simulink model "model4_2"  (R2024a)
settings: Solver=FixedStepAuto  StartTime=0.0  StopTime=36000  FixedStep=0.1  RelTol=1e-3
(part 1 of 7)
settings Model: Creator=rigel  LastModifiedBy=rigel

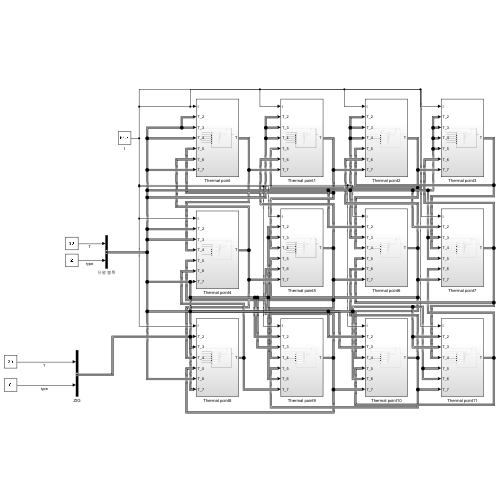
[thumbnail: Simulink's stored preview of the top-level diagram]
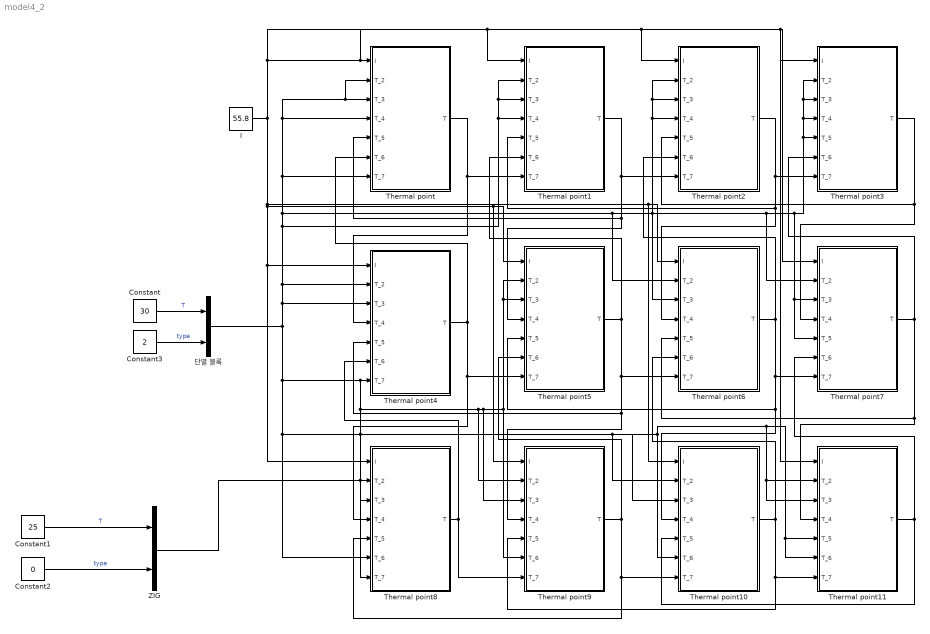
== system model4_2 ==
  Constant : Constant  Value=30
  Constant1 : Constant  Value=25
  Constant2 : Constant  Value=0
  Constant3 : Constant  Value=2
  I : Constant  Value=55.8
  Thermal point : Subsystem
  Thermal point1 : Subsystem
  Thermal point10 : Subsystem
  Thermal point11 : Subsystem
  Thermal point2 : Subsystem
  Thermal point3 : Subsystem
  Thermal point4 : Subsystem
  Thermal point5 : Subsystem
  Thermal point6 : Subsystem
  Thermal point7 : Subsystem
  Thermal point8 : Subsystem
  Thermal point9 : Subsystem
  ZIG : BusCreator  Inputs=2
  단열 블록 : BusCreator  Inputs=2
  wires:
  Constant1/1 -> ZIG/1  "T"
  Constant2/1 -> ZIG/2  "type"
  Constant/1 -> 단열 블록/1  "T"
  Constant3/1 -> 단열 블록/2  "type"
  Thermal point1/1(T) -> Thermal point2/7(T_7), Thermal point5/4(T_4), Thermal point/5(T_5)
  Thermal point2/1(T) -> Thermal point3/7(T_7), Thermal point6/4(T_4), Thermal point1/5(T_5)
  Thermal point3/1(T) -> Thermal point7/4(T_4), Thermal point2/5(T_5)
  Thermal point7/1(T) -> Thermal point3/6(T_6), Thermal point11/4(T_4), Thermal point6/5(T_5)
  Thermal point6/1(T) -> Thermal point7/7(T_7), Thermal point10/4(T_4), Thermal point5/5(T_5), Thermal point2/6(T_6)
  Thermal point5/1(T) -> Thermal point1/6(T_6), Thermal point6/7(T_7), Thermal point9/4(T_4), Thermal point4/5(T_5)
  Thermal point9/1(T) -> Thermal point5/6(T_6), Thermal point10/7(T_7), Thermal point8/5(T_5)
  Thermal point10/1(T) -> Thermal point6/6(T_6), Thermal point11/7(T_7), Thermal point9/5(T_5)
  Thermal point11/1(T) -> Thermal point7/6(T_6), Thermal point10/5(T_5)
  Thermal point/1(T) -> Thermal point1/7(T_7), Thermal point4/4(T_4)
  Thermal point4/1(T) -> Thermal point/6(T_6), Thermal point5/7(T_7), Thermal point8/4(T_4)
  Thermal point8/1(T) -> Thermal point9/7(T_7), Thermal point4/6(T_6)
  단열 블록/1 -> Thermal point8/6(T_6), Thermal point11/6(T_6), Thermal point11/5(T_5), Thermal point11/2(T_2), Thermal point11/3(T_3), Thermal point10/6(T_6), Thermal point10/3(T_3), Thermal point10/2(T_2), Thermal point8/7(T_7), Thermal point5/2(T_2), Thermal point5/3(T_3), Thermal point9/6(T_6), Thermal point9/3(T_3), Thermal point9/2(T_2), Thermal point4/7(T_7), Thermal point7/5(T_5), Thermal point7/3(T_3), Thermal point3/5(T_5), Thermal point3/4(T_4), Thermal point3/3(T_3), Thermal point3/2(T_2), Thermal point7/2(T_2), Thermal point6/3(T_3), Thermal point2/4(T_4), Thermal point2/3(T_3), Thermal point2/2(T_2), Thermal point6/2(T_2), Thermal point/2(T_2), Thermal point/3(T_3), Thermal point/4(T_4), Thermal point/7(T_7), Thermal point1/4(T_4), Thermal point1/3(T_3), Thermal point1/2(T_2), Thermal point4/2(T_2), Thermal point4/3(T_3)
  I/1 -> Thermal point11/1(I), Thermal point7/1(I), Thermal point3/1(I), Thermal point2/1(I), Thermal point1/1(I), Thermal point/1(I), Thermal point10/1(I), Thermal point6/1(I), Thermal point9/1(I), Thermal point5/1(I), Thermal point8/1(I), Thermal point4/1(I)
  ZIG/1 -> Thermal point8/3(T_3), Thermal point8/2(T_2)

== system model4_2/Thermal point ==
  I : Inport
  T_2 : Inport  Port=2
  T_3 : Inport  Port=3
  T_4 : Inport  Port=4
  T_5 : Inport  Port=5
  T_6 : Inport  Port=6
  T_7 : Inport  Port=7
  Sum of Elements : Sum  Inputs=++++++
  Thermal Subsystem : Subsystem
  Thermal trans : Subsystem
  Thermal trans1 : Subsystem
  Thermal trans2 : Subsystem
  Thermal trans3 : Subsystem
  Thermal trans4 : Subsystem
  Thermal trans7 : Subsystem
  Unit Delay : UnitDelay  SampleTime=-1  HasFrameUpgradeWarning=on
  T : Outport
  wires:
  Unit Delay/1 -> Thermal Subsystem/2(Outer Heat)
  Sum of Elements/1 -> Unit Delay/1
  Thermal trans7/1(Outer Heat) -> Sum of Elements/6
  Thermal trans4/1(Outer Heat) -> Sum of Elements/5
  Thermal trans2/1(Outer Heat) -> Sum of Elements/3
  Thermal Subsystem/1(T) -> T/1, Thermal trans/2(Spot T), Thermal trans1/2(Spot T), Thermal trans2/2(Spot T), Thermal trans3/2(Spot T), Thermal trans4/2(Spot T), Thermal trans7/2(Spot T)
  Thermal trans3/1(Outer Heat) -> Sum of Elements/4
  Thermal trans1/1(Outer Heat) -> Sum of Elements/2
  Thermal trans/1(Outer Heat) -> Sum of Elements/1
  I/1 -> Thermal Subsystem/1(I)
  T_2/1 -> Thermal trans/1(Surrounding T)
  T_3/1 -> Thermal trans1/1(Surrounding T)
  T_4/1 -> Thermal trans2/1(Surrounding T)
  T_5/1 -> Thermal trans3/1(Surrounding T)
  T_6/1 -> Thermal trans4/1(Surrounding T)
  T_7/1 -> Thermal trans7/1(Surrounding T)

== system model4_2/Thermal point1 ==
  I : Inport
  T_2 : Inport  Port=2
  T_3 : Inport  Port=3
  T_4 : Inport  Port=4
  T_5 : Inport  Port=5
  T_6 : Inport  Port=6
  T_7 : Inport  Port=7
  Sum of Elements : Sum  Inputs=++++++
  Thermal Subsystem : Subsystem
  Thermal trans : Subsystem
  Thermal trans1 : Subsystem
  Thermal trans2 : Subsystem
  Thermal trans3 : Subsystem
  Thermal trans4 : Subsystem
  Thermal trans7 : Subsystem
  Unit Delay : UnitDelay  SampleTime=-1  HasFrameUpgradeWarning=on
  T : Outport
  wires:
  Unit Delay/1 -> Thermal Subsystem/2(Outer Heat)
  Sum of Elements/1 -> Unit Delay/1
  Thermal trans7/1(Outer Heat) -> Sum of Elements/6
  Thermal trans4/1(Outer Heat) -> Sum of Elements/5
  Thermal trans2/1(Outer Heat) -> Sum of Elements/3
  Thermal Subsystem/1(T) -> T/1, Thermal trans/2(Spot T), Thermal trans1/2(Spot T), Thermal trans2/2(Spot T), Thermal trans3/2(Spot T), Thermal trans4/2(Spot T), Thermal trans7/2(Spot T)
  Thermal trans3/1(Outer Heat) -> Sum of Elements/4
  Thermal trans1/1(Outer Heat) -> Sum of Elements/2
  Thermal trans/1(Outer Heat) -> Sum of Elements/1
  I/1 -> Thermal Subsystem/1(I)
  T_2/1 -> Thermal trans/1(Surrounding T)
  T_3/1 -> Thermal trans1/1(Surrounding T)
  T_4/1 -> Thermal trans2/1(Surrounding T)
  T_5/1 -> Thermal trans3/1(Surrounding T)
  T_6/1 -> Thermal trans4/1(Surrounding T)
  T_7/1 -> Thermal trans7/1(Surrounding T)

== system model4_2/Thermal point10 ==
  I : Inport
  T_2 : Inport  Port=2
  T_3 : Inport  Port=3
  T_4 : Inport  Port=4
  T_5 : Inport  Port=5
  T_6 : Inport  Port=6
  T_7 : Inport  Port=7
  Sum of Elements : Sum  Inputs=++++++
  Thermal Subsystem : Subsystem
  Thermal trans : Subsystem
  Thermal trans1 : Subsystem
  Thermal trans2 : Subsystem
  Thermal trans3 : Subsystem
  Thermal trans4 : Subsystem
  Thermal trans7 : Subsystem
  Unit Delay : UnitDelay  SampleTime=-1  HasFrameUpgradeWarning=on
  T : Outport
  wires:
  Unit Delay/1 -> Thermal Subsystem/2(Outer Heat)
  Sum of Elements/1 -> Unit Delay/1
  Thermal trans7/1(Outer Heat) -> Sum of Elements/6
  Thermal trans4/1(Outer Heat) -> Sum of Elements/5
  Thermal trans2/1(Outer Heat) -> Sum of Elements/3
  Thermal Subsystem/1(T) -> T/1, Thermal trans/2(Spot T), Thermal trans1/2(Spot T), Thermal trans2/2(Spot T), Thermal trans3/2(Spot T), Thermal trans4/2(Spot T), Thermal trans7/2(Spot T)
  Thermal trans3/1(Outer Heat) -> Sum of Elements/4
  Thermal trans1/1(Outer Heat) -> Sum of Elements/2
  Thermal trans/1(Outer Heat) -> Sum of Elements/1
  I/1 -> Thermal Subsystem/1(I)
  T_2/1 -> Thermal trans/1(Surrounding T)
  T_3/1 -> Thermal trans1/1(Surrounding T)
  T_4/1 -> Thermal trans2/1(Surrounding T)
  T_5/1 -> Thermal trans3/1(Surrounding T)
  T_6/1 -> Thermal trans4/1(Surrounding T)
  T_7/1 -> Thermal trans7/1(Surrounding T)

== system model4_2/Thermal point11 ==
  I : Inport
  T_2 : Inport  Port=2
  T_3 : Inport  Port=3
  T_4 : Inport  Port=4
  T_5 : Inport  Port=5
  T_6 : Inport  Port=6
  T_7 : Inport  Port=7
  Sum of Elements : Sum  Inputs=++++++
  Thermal Subsystem : Subsystem
  Thermal trans : Subsystem
  Thermal trans1 : Subsystem
  Thermal trans2 : Subsystem
  Thermal trans3 : Subsystem
  Thermal trans4 : Subsystem
  Thermal trans7 : Subsystem
  Unit Delay : UnitDelay  SampleTime=-1  HasFrameUpgradeWarning=on
  T : Outport
  wires:
  Unit Delay/1 -> Thermal Subsystem/2(Outer Heat)
  Sum of Elements/1 -> Unit Delay/1
  Thermal trans7/1(Outer Heat) -> Sum of Elements/6
  Thermal trans4/1(Outer Heat) -> Sum of Elements/5
  Thermal trans2/1(Outer Heat) -> Sum of Elements/3
  Thermal Subsystem/1(T) -> T/1, Thermal trans/2(Spot T), Thermal trans1/2(Spot T), Thermal trans2/2(Spot T), Thermal trans3/2(Spot T), Thermal trans4/2(Spot T), Thermal trans7/2(Spot T)
  Thermal trans3/1(Outer Heat) -> Sum of Elements/4
  Thermal trans1/1(Outer Heat) -> Sum of Elements/2
  Thermal trans/1(Outer Heat) -> Sum of Elements/1
  I/1 -> Thermal Subsystem/1(I)
  T_2/1 -> Thermal trans/1(Surrounding T)
  T_3/1 -> Thermal trans1/1(Surrounding T)
  T_4/1 -> Thermal trans2/1(Surrounding T)
  T_5/1 -> Thermal trans3/1(Surrounding T)
  T_6/1 -> Thermal trans4/1(Surrounding T)
  T_7/1 -> Thermal trans7/1(Surrounding T)

== system model4_2/Thermal point2 ==
  I : Inport
  T_2 : Inport  Port=2
  T_3 : Inport  Port=3
  T_4 : Inport  Port=4
  T_5 : Inport  Port=5
  T_6 : Inport  Port=6
  T_7 : Inport  Port=7
  Sum of Elements : Sum  Inputs=++++++
  Thermal Subsystem : Subsystem
  Thermal trans : Subsystem
  Thermal trans1 : Subsystem
  Thermal trans2 : Subsystem
  Thermal trans3 : Subsystem
  Thermal trans4 : Subsystem
  Thermal trans7 : Subsystem
  Unit Delay : UnitDelay  SampleTime=-1  HasFrameUpgradeWarning=on
  T : Outport
  wires:
  Unit Delay/1 -> Thermal Subsystem/2(Outer Heat)
  Sum of Elements/1 -> Unit Delay/1
  Thermal trans7/1(Outer Heat) -> Sum of Elements/6
  Thermal trans4/1(Outer Heat) -> Sum of Elements/5
  Thermal trans2/1(Outer Heat) -> Sum of Elements/3
  Thermal Subsystem/1(T) -> T/1, Thermal trans/2(Spot T), Thermal trans1/2(Spot T), Thermal trans2/2(Spot T), Thermal trans3/2(Spot T), Thermal trans4/2(Spot T), Thermal trans7/2(Spot T)
  Thermal trans3/1(Outer Heat) -> Sum of Elements/4
  Thermal trans1/1(Outer Heat) -> Sum of Elements/2
  Thermal trans/1(Outer Heat) -> Sum of Elements/1
  I/1 -> Thermal Subsystem/1(I)
  T_2/1 -> Thermal trans/1(Surrounding T)
  T_3/1 -> Thermal trans1/1(Surrounding T)
  T_4/1 -> Thermal trans2/1(Surrounding T)
  T_5/1 -> Thermal trans3/1(Surrounding T)
  T_6/1 -> Thermal trans4/1(Surrounding T)
  T_7/1 -> Thermal trans7/1(Surrounding T)

== system model4_2/Thermal point3 ==
  I : Inport
  T_2 : Inport  Port=2
  T_3 : Inport  Port=3
  T_4 : Inport  Port=4
  T_5 : Inport  Port=5
  T_6 : Inport  Port=6
  T_7 : Inport  Port=7
  Sum of Elements : Sum  Inputs=++++++
  Thermal Subsystem : Subsystem
  Thermal trans : Subsystem
  Thermal trans1 : Subsystem
  Thermal trans2 : Subsystem
  Thermal trans3 : Subsystem
  Thermal trans4 : Subsystem
  Thermal trans7 : Subsystem
  Unit Delay : UnitDelay  SampleTime=-1  HasFrameUpgradeWarning=on
  T : Outport
  wires:
  Unit Delay/1 -> Thermal Subsystem/2(Outer Heat)
  Sum of Elements/1 -> Unit Delay/1
  Thermal trans7/1(Outer Heat) -> Sum of Elements/6
  Thermal trans4/1(Outer Heat) -> Sum of Elements/5
  Thermal trans2/1(Outer Heat) -> Sum of Elements/3
  Thermal Subsystem/1(T) -> T/1, Thermal trans/2(Spot T), Thermal trans1/2(Spot T), Thermal trans2/2(Spot T), Thermal trans3/2(Spot T), Thermal trans4/2(Spot T), Thermal trans7/2(Spot T)
  Thermal trans3/1(Outer Heat) -> Sum of Elements/4
  Thermal trans1/1(Outer Heat) -> Sum of Elements/2
  Thermal trans/1(Outer Heat) -> Sum of Elements/1
  I/1 -> Thermal Subsystem/1(I)
  T_2/1 -> Thermal trans/1(Surrounding T)
  T_3/1 -> Thermal trans1/1(Surrounding T)
  T_4/1 -> Thermal trans2/1(Surrounding T)
  T_5/1 -> Thermal trans3/1(Surrounding T)
  T_6/1 -> Thermal trans4/1(Surrounding T)
  T_7/1 -> Thermal trans7/1(Surrounding T)

== system model4_2/Thermal point4 ==
  I : Inport
  T_2 : Inport  Port=2
  T_3 : Inport  Port=3
  T_4 : Inport  Port=4
  T_5 : Inport  Port=5
  T_6 : Inport  Port=6
  T_7 : Inport  Port=7
  Sum of Elements : Sum  Inputs=++++++
  Thermal Subsystem : Subsystem
  Thermal trans : Subsystem
  Thermal trans1 : Subsystem
  Thermal trans2 : Subsystem
  Thermal trans3 : Subsystem
  Thermal trans4 : Subsystem
  Thermal trans7 : Subsystem
  Unit Delay : UnitDelay  SampleTime=-1  HasFrameUpgradeWarning=on
  T : Outport
  wires:
  Unit Delay/1 -> Thermal Subsystem/2(Outer Heat)
  Sum of Elements/1 -> Unit Delay/1
  Thermal trans7/1(Outer Heat) -> Sum of Elements/6
  Thermal trans4/1(Outer Heat) -> Sum of Elements/5
  Thermal trans2/1(Outer Heat) -> Sum of Elements/3
  Thermal Subsystem/1(T) -> T/1, Thermal trans/2(Spot T), Thermal trans1/2(Spot T), Thermal trans2/2(Spot T), Thermal trans3/2(Spot T), Thermal trans4/2(Spot T), Thermal trans7/2(Spot T)
  Thermal trans3/1(Outer Heat) -> Sum of Elements/4
  Thermal trans1/1(Outer Heat) -> Sum of Elements/2
  Thermal trans/1(Outer Heat) -> Sum of Elements/1
  I/1 -> Thermal Subsystem/1(I)
  T_2/1 -> Thermal trans/1(Surrounding T)
  T_3/1 -> Thermal trans1/1(Surrounding T)
  T_4/1 -> Thermal trans2/1(Surrounding T)
  T_5/1 -> Thermal trans3/1(Surrounding T)
  T_6/1 -> Thermal trans4/1(Surrounding T)
  T_7/1 -> Thermal trans7/1(Surrounding T)

== system model4_2/Thermal point5 ==
  I : Inport
  T_2 : Inport  Port=2
  T_3 : Inport  Port=3
  T_4 : Inport  Port=4
  T_5 : Inport  Port=5
  T_6 : Inport  Port=6
  T_7 : Inport  Port=7
  Sum of Elements : Sum  Inputs=++++++
  Thermal Subsystem : Subsystem
  Thermal trans : Subsystem
  Thermal trans1 : Subsystem
  Thermal trans2 : Subsystem
  Thermal trans3 : Subsystem
  Thermal trans4 : Subsystem
  Thermal trans7 : Subsystem
  Unit Delay : UnitDelay  SampleTime=-1  HasFrameUpgradeWarning=on
  T : Outport
  wires:
  Unit Delay/1 -> Thermal Subsystem/2(Outer Heat)
  Sum of Elements/1 -> Unit Delay/1
  Thermal trans7/1(Outer Heat) -> Sum of Elements/6
  Thermal trans4/1(Outer Heat) -> Sum of Elements/5
  Thermal trans2/1(Outer Heat) -> Sum of Elements/3
  Thermal Subsystem/1(T) -> T/1, Thermal trans/2(Spot T), Thermal trans1/2(Spot T), Thermal trans2/2(Spot T), Thermal trans3/2(Spot T), Thermal trans4/2(Spot T), Thermal trans7/2(Spot T)
  Thermal trans3/1(Outer Heat) -> Sum of Elements/4
  Thermal trans1/1(Outer Heat) -> Sum of Elements/2
  Thermal trans/1(Outer Heat) -> Sum of Elements/1
  I/1 -> Thermal Subsystem/1(I)
  T_2/1 -> Thermal trans/1(Surrounding T)
  T_3/1 -> Thermal trans1/1(Surrounding T)
  T_4/1 -> Thermal trans2/1(Surrounding T)
  T_5/1 -> Thermal trans3/1(Surrounding T)
  T_6/1 -> Thermal trans4/1(Surrounding T)
  T_7/1 -> Thermal trans7/1(Surrounding T)

== system model4_2/Thermal point6 ==
  I : Inport
  T_2 : Inport  Port=2
  T_3 : Inport  Port=3
  T_4 : Inport  Port=4
  T_5 : Inport  Port=5
  T_6 : Inport  Port=6
  T_7 : Inport  Port=7
  Sum of Elements : Sum  Inputs=++++++
  Thermal Subsystem : Subsystem
  Thermal trans : Subsystem
  Thermal trans1 : Subsystem
  Thermal trans2 : Subsystem
  Thermal trans3 : Subsystem
  Thermal trans4 : Subsystem
  Thermal trans7 : Subsystem
  Unit Delay : UnitDelay  SampleTime=-1  HasFrameUpgradeWarning=on
  T : Outport
  wires:
  Unit Delay/1 -> Thermal Subsystem/2(Outer Heat)
  Sum of Elements/1 -> Unit Delay/1
  Thermal trans7/1(Outer Heat) -> Sum of Elements/6
  Thermal trans4/1(Outer Heat) -> Sum of Elements/5
  Thermal trans2/1(Outer Heat) -> Sum of Elements/3
  Thermal Subsystem/1(T) -> T/1, Thermal trans/2(Spot T), Thermal trans1/2(Spot T), Thermal trans2/2(Spot T), Thermal trans3/2(Spot T), Thermal trans4/2(Spot T), Thermal trans7/2(Spot T)
  Thermal trans3/1(Outer Heat) -> Sum of Elements/4
  Thermal trans1/1(Outer Heat) -> Sum of Elements/2
  Thermal trans/1(Outer Heat) -> Sum of Elements/1
  I/1 -> Thermal Subsystem/1(I)
  T_2/1 -> Thermal trans/1(Surrounding T)
  T_3/1 -> Thermal trans1/1(Surrounding T)
  T_4/1 -> Thermal trans2/1(Surrounding T)
  T_5/1 -> Thermal trans3/1(Surrounding T)
  T_6/1 -> Thermal trans4/1(Surrounding T)
  T_7/1 -> Thermal trans7/1(Surrounding T)

== system model4_2/Thermal point7 ==
  I : Inport
  T_2 : Inport  Port=2
  T_3 : Inport  Port=3
  T_4 : Inport  Port=4
  T_5 : Inport  Port=5
  T_6 : Inport  Port=6
  T_7 : Inport  Port=7
  Sum of Elements : Sum  Inputs=++++++
  Thermal Subsystem : Subsystem
  Thermal trans : Subsystem
  Thermal trans1 : Subsystem
  Thermal trans2 : Subsystem
  Thermal trans3 : Subsystem
  Thermal trans4 : Subsystem
  Thermal trans7 : Subsystem
  Unit Delay : UnitDelay  SampleTime=-1  HasFrameUpgradeWarning=on
  T : Outport
  wires:
  Unit Delay/1 -> Thermal Subsystem/2(Outer Heat)
  Sum of Elements/1 -> Unit Delay/1
  Thermal trans7/1(Outer Heat) -> Sum of Elements/6
  Thermal trans4/1(Outer Heat) -> Sum of Elements/5
  Thermal trans2/1(Outer Heat) -> Sum of Elements/3
  Thermal Subsystem/1(T) -> T/1, Thermal trans/2(Spot T), Thermal trans1/2(Spot T), Thermal trans2/2(Spot T), Thermal trans3/2(Spot T), Thermal trans4/2(Spot T), Thermal trans7/2(Spot T)
  Thermal trans3/1(Outer Heat) -> Sum of Elements/4
  Thermal trans1/1(Outer Heat) -> Sum of Elements/2
  Thermal trans/1(Outer Heat) -> Sum of Elements/1
  I/1 -> Thermal Subsystem/1(I)
  T_2/1 -> Thermal trans/1(Surrounding T)
  T_3/1 -> Thermal trans1/1(Surrounding T)
  T_4/1 -> Thermal trans2/1(Surrounding T)
  T_5/1 -> Thermal trans3/1(Surrounding T)
  T_6/1 -> Thermal trans4/1(Surrounding T)
  T_7/1 -> Thermal trans7/1(Surrounding T)

== system model4_2/Thermal point8 ==
  I : Inport
  T_2 : Inport  Port=2
  T_3 : Inport  Port=3
  T_4 : Inport  Port=4
  T_5 : Inport  Port=5
  T_6 : Inport  Port=6
  T_7 : Inport  Port=7
  Sum of Elements : Sum  Inputs=++++++
  Thermal Subsystem : Subsystem
  Thermal trans : Subsystem
  Thermal trans1 : Subsystem
  Thermal trans2 : Subsystem
  Thermal trans3 : Subsystem
  Thermal trans4 : Subsystem
  Thermal trans7 : Subsystem
  Unit Delay : UnitDelay  SampleTime=-1  HasFrameUpgradeWarning=on
  T : Outport
  wires:
  Unit Delay/1 -> Thermal Subsystem/2(Outer Heat)
  Sum of Elements/1 -> Unit Delay/1
  Thermal trans7/1(Outer Heat) -> Sum of Elements/6
  Thermal trans4/1(Outer Heat) -> Sum of Elements/5
  Thermal trans2/1(Outer Heat) -> Sum of Elements/3
  Thermal Subsystem/1(T) -> T/1, Thermal trans/2(Spot T), Thermal trans1/2(Spot T), Thermal trans2/2(Spot T), Thermal trans3/2(Spot T), Thermal trans4/2(Spot T), Thermal trans7/2(Spot T)
  Thermal trans3/1(Outer Heat) -> Sum of Elements/4
  Thermal trans1/1(Outer Heat) -> Sum of Elements/2
  Thermal trans/1(Outer Heat) -> Sum of Elements/1
  I/1 -> Thermal Subsystem/1(I)
  T_2/1 -> Thermal trans/1(Surrounding T)
  T_3/1 -> Thermal trans1/1(Surrounding T)
  T_4/1 -> Thermal trans2/1(Surrounding T)
  T_5/1 -> Thermal trans3/1(Surrounding T)
  T_6/1 -> Thermal trans4/1(Surrounding T)
  T_7/1 -> Thermal trans7/1(Surrounding T)

== system model4_2/Thermal point9 ==
  I : Inport
  T_2 : Inport  Port=2
  T_3 : Inport  Port=3
  T_4 : Inport  Port=4
  T_5 : Inport  Port=5
  T_6 : Inport  Port=6
  T_7 : Inport  Port=7
  Sum of Elements : Sum  Inputs=++++++
  Thermal Subsystem : Subsystem
  Thermal trans : Subsystem
  Thermal trans1 : Subsystem
  Thermal trans2 : Subsystem
  Thermal trans3 : Subsystem
  Thermal trans4 : Subsystem
  Thermal trans7 : Subsystem
  Unit Delay : UnitDelay  SampleTime=-1  HasFrameUpgradeWarning=on
  T : Outport
  wires:
  Unit Delay/1 -> Thermal Subsystem/2(Outer Heat)
  Sum of Elements/1 -> Unit Delay/1
  Thermal trans7/1(Outer Heat) -> Sum of Elements/6
  Thermal trans4/1(Outer Heat) -> Sum of Elements/5
  Thermal trans2/1(Outer Heat) -> Sum of Elements/3
  Thermal Subsystem/1(T) -> T/1, Thermal trans/2(Spot T), Thermal trans1/2(Spot T), Thermal trans2/2(Spot T), Thermal trans3/2(Spot T), Thermal trans4/2(Spot T), Thermal trans7/2(Spot T)
  Thermal trans3/1(Outer Heat) -> Sum of Elements/4
  Thermal trans1/1(Outer Heat) -> Sum of Elements/2
  Thermal trans/1(Outer Heat) -> Sum of Elements/1
  I/1 -> Thermal Subsystem/1(I)
  T_2/1 -> Thermal trans/1(Surrounding T)
  T_3/1 -> Thermal trans1/1(Surrounding T)
  T_4/1 -> Thermal trans2/1(Surrounding T)
  T_5/1 -> Thermal trans3/1(Surrounding T)
  T_6/1 -> Thermal trans4/1(Surrounding T)
  T_7/1 -> Thermal trans7/1(Surrounding T)

== system model4_2/Thermal point/Thermal Subsystem ==
  I : Inport
  Outer Heat : Inport  Port=2
  Bus Creator : BusCreator  Inputs=2
  Electrical model : Subsystem
  Heat model : Subsystem
  Parameter : Subsystem
  "T, SOC" : Subsystem
  Unit Delay : UnitDelay  SampleTime=-1  HasFrameUpgradeWarning=on
  cond : Constant  Value=0
  T : Outport
  wires:
  Parameter/2(Non Varing Parameters) -> Electrical model/3(Non Varing Parameters), Heat model/5(Non Varing Parameters)
  "T, SOC"/1(Varing parameters) -> Electrical model/2(Varing parameters), Heat model/4(Varing parameters)
  I/1 -> Heat model/3(I), Electrical model/1(I)
  Electrical model/2(SOC) -> Parameter/2(SOC)
  Electrical model/1(voltage) -> Heat model/2(voltage)
  Parameter/1("T, SOC") -> Heat model/6("T, SOC"), "T, SOC"/1("T, SOC")
  Outer Heat/1 -> Heat model/1(Outer Heat)
  Heat model/1(T) -> Bus Creator/1, Parameter/1(T)
  Bus Creator/1 -> T/1
  cond/1 -> Unit Delay/1  "type"
  Unit Delay/1 -> Bus Creator/2  "type"

== system model4_2/Thermal point/Thermal trans ==
  Surrounding T : Inport
  Spot T : Inport  Port=2
  Bus Selector : BusSelector  OutputSignals=T,type
  Bus Selector1 : BusSelector  OutputSignals=T
  Heat Trans : MATLAB Function  TreatAsAtomicUnit=on
  Scope : Scope
  Scope2 : Scope
  Scope3 : Scope
  Outer Heat : Outport
  wires:
  Heat Trans/1(Outer_Heat) -> Scope/1, Outer Heat/1
  Bus Selector/1 -> Scope2/1, Heat Trans/2(Surrounding_T)  "<T>"
  Bus Selector/2 -> Heat Trans/3(type)  "<type>"
  Bus Selector1/1 -> Scope3/1, Heat Trans/1(Inner_T)  "<T>"
  Spot T/1 -> Bus Selector1/1
  Surrounding T/1 -> Bus Selector/1

== system model4_2/Thermal point/Thermal trans1 ==
  Surrounding T : Inport
  Spot T : Inport  Port=2
  Bus Selector : BusSelector  OutputSignals=T,type
  Bus Selector1 : BusSelector  OutputSignals=T
  Heat Trans : MATLAB Function  TreatAsAtomicUnit=on
  Scope : Scope
  Scope2 : Scope
  Scope3 : Scope
  Outer Heat : Outport
  wires:
  Heat Trans/1(Outer_Heat) -> Scope/1, Outer Heat/1
  Bus Selector/1 -> Scope2/1, Heat Trans/2(Surrounding_T)  "<T>"
  Bus Selector/2 -> Heat Trans/3(type)  "<type>"
  Bus Selector1/1 -> Scope3/1, Heat Trans/1(Inner_T)  "<T>"
  Spot T/1 -> Bus Selector1/1
  Surrounding T/1 -> Bus Selector/1

== system model4_2/Thermal point/Thermal trans2 ==
  Surrounding T : Inport
  Spot T : Inport  Port=2
  Bus Selector : BusSelector  OutputSignals=T,type
  Bus Selector1 : BusSelector  OutputSignals=T
  Heat Trans : MATLAB Function  TreatAsAtomicUnit=on
  Scope : Scope
  Scope2 : Scope
  Scope3 : Scope
  Outer Heat : Outport
  wires:
  Heat Trans/1(Outer_Heat) -> Scope/1, Outer Heat/1
  Bus Selector/1 -> Scope2/1, Heat Trans/2(Surrounding_T)  "<T>"
  Bus Selector/2 -> Heat Trans/3(type)  "<type>"
  Bus Selector1/1 -> Scope3/1, Heat Trans/1(Inner_T)  "<T>"
  Spot T/1 -> Bus Selector1/1
  Surrounding T/1 -> Bus Selector/1

== system model4_2/Thermal point/Thermal trans3 ==
  Surrounding T : Inport
  Spot T : Inport  Port=2
  Bus Selector : BusSelector  OutputSignals=T,type
  Bus Selector1 : BusSelector  OutputSignals=T
  Heat Trans : MATLAB Function  TreatAsAtomicUnit=on
  Scope : Scope
  Scope2 : Scope
  Scope3 : Scope
  Outer Heat : Outport
  wires:
  Heat Trans/1(Outer_Heat) -> Scope/1, Outer Heat/1
  Bus Selector/1 -> Scope2/1, Heat Trans/2(Surrounding_T)  "<T>"
  Bus Selector/2 -> Heat Trans/3(type)  "<type>"
  Bus Selector1/1 -> Scope3/1, Heat Trans/1(Inner_T)  "<T>"
  Spot T/1 -> Bus Selector1/1
  Surrounding T/1 -> Bus Selector/1

== system model4_2/Thermal point/Thermal trans4 ==
  Surrounding T : Inport
  Spot T : Inport  Port=2
  Bus Selector : BusSelector  OutputSignals=T,type
  Bus Selector1 : BusSelector  OutputSignals=T
  Heat Trans : MATLAB Function  TreatAsAtomicUnit=on
  Scope : Scope
  Scope2 : Scope
  Scope3 : Scope
  Outer Heat : Outport
  wires:
  Heat Trans/1(Outer_Heat) -> Scope/1, Outer Heat/1
  Bus Selector/1 -> Scope2/1, Heat Trans/2(Surrounding_T)  "<T>"
  Bus Selector/2 -> Heat Trans/3(type)  "<type>"
  Bus Selector1/1 -> Scope3/1, Heat Trans/1(Inner_T)  "<T>"
  Spot T/1 -> Bus Selector1/1
  Surrounding T/1 -> Bus Selector/1

== system model4_2/Thermal point/Thermal trans7 ==
  Surrounding T : Inport
  Spot T : Inport  Port=2
  Bus Selector : BusSelector  OutputSignals=T,type
  Bus Selector1 : BusSelector  OutputSignals=T
  Heat Trans : MATLAB Function  TreatAsAtomicUnit=on
  Scope : Scope
  Scope2 : Scope
  Scope3 : Scope
  Outer Heat : Outport
  wires:
  Heat Trans/1(Outer_Heat) -> Scope/1, Outer Heat/1
  Bus Selector/1 -> Scope2/1, Heat Trans/2(Surrounding_T)  "<T>"
  Bus Selector1/1 -> Scope3/1, Heat Trans/1(Inner_T)  "<T>"
  Spot T/1 -> Bus Selector1/1
  Surrounding T/1 -> Bus Selector/1
  Bus Selector/2 -> Heat Trans/3(type)  "<type>"

== system model4_2/Thermal point1/Thermal Subsystem ==
  I : Inport
  Outer Heat : Inport  Port=2
  Bus Creator : BusCreator  Inputs=2
  Electrical model : Subsystem
  Heat model : Subsystem
  Parameter : Subsystem
  "T, SOC" : Subsystem
  Unit Delay : UnitDelay  SampleTime=-1  HasFrameUpgradeWarning=on
  cond : Constant  Value=0
  T : Outport
  wires:
  Parameter/2(Non Varing Parameters) -> Electrical model/3(Non Varing Parameters), Heat model/5(Non Varing Parameters)
  "T, SOC"/1(Varing parameters) -> Electrical model/2(Varing parameters), Heat model/4(Varing parameters)
  I/1 -> Heat model/3(I), Electrical model/1(I)
  Electrical model/2(SOC) -> Parameter/2(SOC)
  Electrical model/1(voltage) -> Heat model/2(voltage)
  Parameter/1("T, SOC") -> Heat model/6("T, SOC"), "T, SOC"/1("T, SOC")
  Outer Heat/1 -> Heat model/1(Outer Heat)
  Heat model/1(T) -> Bus Creator/1, Parameter/1(T)
  Bus Creator/1 -> T/1
  cond/1 -> Unit Delay/1  "type"
  Unit Delay/1 -> Bus Creator/2  "type"

== system model4_2/Thermal point1/Thermal trans ==
  Surrounding T : Inport
  Spot T : Inport  Port=2
  Bus Selector : BusSelector  OutputSignals=T,type
  Bus Selector1 : BusSelector  OutputSignals=T
  Heat Trans : MATLAB Function  TreatAsAtomicUnit=on
  Scope : Scope
  Scope2 : Scope
  Scope3 : Scope
  Outer Heat : Outport
  wires:
  Heat Trans/1(Outer_Heat) -> Scope/1, Outer Heat/1
  Bus Selector/1 -> Scope2/1, Heat Trans/2(Surrounding_T)  "<T>"
  Bus Selector/2 -> Heat Trans/3(type)  "<type>"
  Bus Selector1/1 -> Scope3/1, Heat Trans/1(Inner_T)  "<T>"
  Spot T/1 -> Bus Selector1/1
  Surrounding T/1 -> Bus Selector/1

== system model4_2/Thermal point1/Thermal trans1 ==
  Surrounding T : Inport
  Spot T : Inport  Port=2
  Bus Selector : BusSelector  OutputSignals=T,type
  Bus Selector1 : BusSelector  OutputSignals=T
  Heat Trans : MATLAB Function  TreatAsAtomicUnit=on
  Scope : Scope
  Scope2 : Scope
  Scope3 : Scope
  Outer Heat : Outport
  wires:
  Heat Trans/1(Outer_Heat) -> Scope/1, Outer Heat/1
  Bus Selector/1 -> Scope2/1, Heat Trans/2(Surrounding_T)  "<T>"
  Bus Selector/2 -> Heat Trans/3(type)  "<type>"
  Bus Selector1/1 -> Scope3/1, Heat Trans/1(Inner_T)  "<T>"
  Spot T/1 -> Bus Selector1/1
  Surrounding T/1 -> Bus Selector/1

== system model4_2/Thermal point1/Thermal trans2 ==
  Surrounding T : Inport
  Spot T : Inport  Port=2
  Bus Selector : BusSelector  OutputSignals=T,type
  Bus Selector1 : BusSelector  OutputSignals=T
  Heat Trans : MATLAB Function  TreatAsAtomicUnit=on
  Scope : Scope
  Scope2 : Scope
  Scope3 : Scope
  Outer Heat : Outport
  wires:
  Heat Trans/1(Outer_Heat) -> Scope/1, Outer Heat/1
  Bus Selector/1 -> Scope2/1, Heat Trans/2(Surrounding_T)  "<T>"
  Bus Selector/2 -> Heat Trans/3(type)  "<type>"
  Bus Selector1/1 -> Scope3/1, Heat Trans/1(Inner_T)  "<T>"
  Spot T/1 -> Bus Selector1/1
  Surrounding T/1 -> Bus Selector/1

== system model4_2/Thermal point1/Thermal trans3 ==
  Surrounding T : Inport
  Spot T : Inport  Port=2
  Bus Selector : BusSelector  OutputSignals=T,type
  Bus Selector1 : BusSelector  OutputSignals=T
  Heat Trans : MATLAB Function  TreatAsAtomicUnit=on
  Scope : Scope
  Scope2 : Scope
  Scope3 : Scope
  Outer Heat : Outport
  wires:
  Heat Trans/1(Outer_Heat) -> Scope/1, Outer Heat/1
  Bus Selector/1 -> Scope2/1, Heat Trans/2(Surrounding_T)  "<T>"
  Bus Selector/2 -> Heat Trans/3(type)  "<type>"
  Bus Selector1/1 -> Scope3/1, Heat Trans/1(Inner_T)  "<T>"
  Spot T/1 -> Bus Selector1/1
  Surrounding T/1 -> Bus Selector/1

== system model4_2/Thermal point1/Thermal trans4 ==
  Surrounding T : Inport
  Spot T : Inport  Port=2
  Bus Selector : BusSelector  OutputSignals=T,type
  Bus Selector1 : BusSelector  OutputSignals=T
  Heat Trans : MATLAB Function  TreatAsAtomicUnit=on
  Scope : Scope
  Scope2 : Scope
  Scope3 : Scope
  Outer Heat : Outport
  wires:
  Heat Trans/1(Outer_Heat) -> Scope/1, Outer Heat/1
  Bus Selector/1 -> Scope2/1, Heat Trans/2(Surrounding_T)  "<T>"
  Bus Selector/2 -> Heat Trans/3(type)  "<type>"
  Bus Selector1/1 -> Scope3/1, Heat Trans/1(Inner_T)  "<T>"
  Spot T/1 -> Bus Selector1/1
  Surrounding T/1 -> Bus Selector/1

== system model4_2/Thermal point1/Thermal trans7 ==
  Surrounding T : Inport
  Spot T : Inport  Port=2
  Bus Selector : BusSelector  OutputSignals=T,type
  Bus Selector1 : BusSelector  OutputSignals=T
  Heat Trans : MATLAB Function  TreatAsAtomicUnit=on
  Scope : Scope
  Scope2 : Scope
  Scope3 : Scope
  Outer Heat : Outport
  wires:
  Heat Trans/1(Outer_Heat) -> Scope/1, Outer Heat/1
  Bus Selector/1 -> Scope2/1, Heat Trans/2(Surrounding_T)  "<T>"
  Bus Selector1/1 -> Scope3/1, Heat Trans/1(Inner_T)  "<T>"
  Spot T/1 -> Bus Selector1/1
  Surrounding T/1 -> Bus Selector/1
  Bus Selector/2 -> Heat Trans/3(type)  "<type>"

== system model4_2/Thermal point10/Thermal Subsystem ==
  I : Inport
  Outer Heat : Inport  Port=2
  Bus Creator : BusCreator  Inputs=2
  Electrical model : Subsystem
  Heat model : Subsystem
  Parameter : Subsystem
  "T, SOC" : Subsystem
  Unit Delay : UnitDelay  SampleTime=-1  HasFrameUpgradeWarning=on
  cond : Constant  Value=0
  T : Outport
  wires:
  Parameter/2(Non Varing Parameters) -> Electrical model/3(Non Varing Parameters), Heat model/5(Non Varing Parameters)
  "T, SOC"/1(Varing parameters) -> Electrical model/2(Varing parameters), Heat model/4(Varing parameters)
  I/1 -> Heat model/3(I), Electrical model/1(I)
  Electrical model/2(SOC) -> Parameter/2(SOC)
  Electrical model/1(voltage) -> Heat model/2(voltage)
  Parameter/1("T, SOC") -> Heat model/6("T, SOC"), "T, SOC"/1("T, SOC")
  Outer Heat/1 -> Heat model/1(Outer Heat)
  Heat model/1(T) -> Bus Creator/1, Parameter/1(T)
  Bus Creator/1 -> T/1
  cond/1 -> Unit Delay/1  "type"
  Unit Delay/1 -> Bus Creator/2  "type"

== system model4_2/Thermal point10/Thermal trans ==
  Surrounding T : Inport
  Spot T : Inport  Port=2
  Bus Selector : BusSelector  OutputSignals=T,type
  Bus Selector1 : BusSelector  OutputSignals=T
  Heat Trans : MATLAB Function  TreatAsAtomicUnit=on
  Scope : Scope
  Scope2 : Scope
  Scope3 : Scope
  Outer Heat : Outport
  wires:
  Heat Trans/1(Outer_Heat) -> Scope/1, Outer Heat/1
  Bus Selector/1 -> Scope2/1, Heat Trans/2(Surrounding_T)  "<T>"
  Bus Selector/2 -> Heat Trans/3(type)  "<type>"
  Bus Selector1/1 -> Scope3/1, Heat Trans/1(Inner_T)  "<T>"
  Spot T/1 -> Bus Selector1/1
  Surrounding T/1 -> Bus Selector/1

== system model4_2/Thermal point10/Thermal trans1 ==
  Surrounding T : Inport
  Spot T : Inport  Port=2
  Bus Selector : BusSelector  OutputSignals=T,type
  Bus Selector1 : BusSelector  OutputSignals=T
  Heat Trans : MATLAB Function  TreatAsAtomicUnit=on
  Scope : Scope
  Scope2 : Scope
  Scope3 : Scope
  Outer Heat : Outport
  wires:
  Heat Trans/1(Outer_Heat) -> Scope/1, Outer Heat/1
  Bus Selector/1 -> Scope2/1, Heat Trans/2(Surrounding_T)  "<T>"
  Bus Selector/2 -> Heat Trans/3(type)  "<type>"
  Bus Selector1/1 -> Scope3/1, Heat Trans/1(Inner_T)  "<T>"
  Spot T/1 -> Bus Selector1/1
  Surrounding T/1 -> Bus Selector/1

== system model4_2/Thermal point10/Thermal trans2 ==
  Surrounding T : Inport
  Spot T : Inport  Port=2
  Bus Selector : BusSelector  OutputSignals=T,type
  Bus Selector1 : BusSelector  OutputSignals=T
  Heat Trans : MATLAB Function  TreatAsAtomicUnit=on
  Scope : Scope
  Scope2 : Scope
  Scope3 : Scope
  Outer Heat : Outport
  wires:
  Heat Trans/1(Outer_Heat) -> Scope/1, Outer Heat/1
  Bus Selector/1 -> Scope2/1, Heat Trans/2(Surrounding_T)  "<T>"
  Bus Selector/2 -> Heat Trans/3(type)  "<type>"
  Bus Selector1/1 -> Scope3/1, Heat Trans/1(Inner_T)  "<T>"
  Spot T/1 -> Bus Selector1/1
  Surrounding T/1 -> Bus Selector/1

== system model4_2/Thermal point10/Thermal trans3 ==
  Surrounding T : Inport
  Spot T : Inport  Port=2
  Bus Selector : BusSelector  OutputSignals=T,type
  Bus Selector1 : BusSelector  OutputSignals=T
  Heat Trans : MATLAB Function  TreatAsAtomicUnit=on
  Scope : Scope
  Scope2 : Scope
  Scope3 : Scope
  Outer Heat : Outport
  wires:
  Heat Trans/1(Outer_Heat) -> Scope/1, Outer Heat/1
  Bus Selector/1 -> Scope2/1, Heat Trans/2(Surrounding_T)  "<T>"
  Bus Selector/2 -> Heat Trans/3(type)  "<type>"
  Bus Selector1/1 -> Scope3/1, Heat Trans/1(Inner_T)  "<T>"
  Spot T/1 -> Bus Selector1/1
  Surrounding T/1 -> Bus Selector/1

== system model4_2/Thermal point10/Thermal trans4 ==
  Surrounding T : Inport
  Spot T : Inport  Port=2
  Bus Selector : BusSelector  OutputSignals=T,type
  Bus Selector1 : BusSelector  OutputSignals=T
  Heat Trans : MATLAB Function  TreatAsAtomicUnit=on
  Scope : Scope
  Scope2 : Scope
  Scope3 : Scope
  Outer Heat : Outport
  wires:
  Heat Trans/1(Outer_Heat) -> Scope/1, Outer Heat/1
  Bus Selector/1 -> Scope2/1, Heat Trans/2(Surrounding_T)  "<T>"
  Bus Selector/2 -> Heat Trans/3(type)  "<type>"
  Bus Selector1/1 -> Scope3/1, Heat Trans/1(Inner_T)  "<T>"
  Spot T/1 -> Bus Selector1/1
  Surrounding T/1 -> Bus Selector/1

== system model4_2/Thermal point10/Thermal trans7 ==
  Surrounding T : Inport
  Spot T : Inport  Port=2
  Bus Selector : BusSelector  OutputSignals=T,type
  Bus Selector1 : BusSelector  OutputSignals=T
  Heat Trans : MATLAB Function  TreatAsAtomicUnit=on
  Scope : Scope
  Scope2 : Scope
  Scope3 : Scope
  Outer Heat : Outport
  wires:
  Heat Trans/1(Outer_Heat) -> Scope/1, Outer Heat/1
  Bus Selector/1 -> Scope2/1, Heat Trans/2(Surrounding_T)  "<T>"
  Bus Selector1/1 -> Scope3/1, Heat Trans/1(Inner_T)  "<T>"
  Spot T/1 -> Bus Selector1/1
  Surrounding T/1 -> Bus Selector/1
  Bus Selector/2 -> Heat Trans/3(type)  "<type>"

== system model4_2/Thermal point11/Thermal Subsystem ==
  I : Inport
  Outer Heat : Inport  Port=2
  Bus Creator : BusCreator  Inputs=2
  Electrical model : Subsystem
  Heat model : Subsystem
  Parameter : Subsystem
  "T, SOC" : Subsystem
  Unit Delay : UnitDelay  SampleTime=-1  HasFrameUpgradeWarning=on
  cond : Constant  Value=0
  T : Outport
  wires:
  Parameter/2(Non Varing Parameters) -> Electrical model/3(Non Varing Parameters), Heat model/5(Non Varing Parameters)
  "T, SOC"/1(Varing parameters) -> Electrical model/2(Varing parameters), Heat model/4(Varing parameters)
  I/1 -> Heat model/3(I), Electrical model/1(I)
  Electrical model/2(SOC) -> Parameter/2(SOC)
  Electrical model/1(voltage) -> Heat model/2(voltage)
  Parameter/1("T, SOC") -> Heat model/6("T, SOC"), "T, SOC"/1("T, SOC")
  Outer Heat/1 -> Heat model/1(Outer Heat)
  Heat model/1(T) -> Bus Creator/1, Parameter/1(T)
  Bus Creator/1 -> T/1
  cond/1 -> Unit Delay/1  "type"
  Unit Delay/1 -> Bus Creator/2  "type"

== system model4_2/Thermal point11/Thermal trans ==
  Surrounding T : Inport
  Spot T : Inport  Port=2
  Bus Selector : BusSelector  OutputSignals=T,type
  Bus Selector1 : BusSelector  OutputSignals=T
  Heat Trans : MATLAB Function  TreatAsAtomicUnit=on
  Scope : Scope
  Scope2 : Scope
  Scope3 : Scope
  Outer Heat : Outport
  wires:
  Heat Trans/1(Outer_Heat) -> Scope/1, Outer Heat/1
  Bus Selector/1 -> Scope2/1, Heat Trans/2(Surrounding_T)  "<T>"
  Bus Selector/2 -> Heat Trans/3(type)  "<type>"
  Bus Selector1/1 -> Scope3/1, Heat Trans/1(Inner_T)  "<T>"
  Spot T/1 -> Bus Selector1/1
  Surrounding T/1 -> Bus Selector/1

== system model4_2/Thermal point11/Thermal trans1 ==
  Surrounding T : Inport
  Spot T : Inport  Port=2
  Bus Selector : BusSelector  OutputSignals=T,type
  Bus Selector1 : BusSelector  OutputSignals=T
  Heat Trans : MATLAB Function  TreatAsAtomicUnit=on
  Scope : Scope
  Scope2 : Scope
  Scope3 : Scope
  Outer Heat : Outport
  wires:
  Heat Trans/1(Outer_Heat) -> Scope/1, Outer Heat/1
  Bus Selector/1 -> Scope2/1, Heat Trans/2(Surrounding_T)  "<T>"
  Bus Selector/2 -> Heat Trans/3(type)  "<type>"
  Bus Selector1/1 -> Scope3/1, Heat Trans/1(Inner_T)  "<T>"
  Spot T/1 -> Bus Selector1/1
  Surrounding T/1 -> Bus Selector/1

== system model4_2/Thermal point11/Thermal trans2 ==
  Surrounding T : Inport
  Spot T : Inport  Port=2
  Bus Selector : BusSelector  OutputSignals=T,type
  Bus Selector1 : BusSelector  OutputSignals=T
  Heat Trans : MATLAB Function  TreatAsAtomicUnit=on
  Scope : Scope
  Scope2 : Scope
  Scope3 : Scope
  Outer Heat : Outport
  wires:
  Heat Trans/1(Outer_Heat) -> Scope/1, Outer Heat/1
  Bus Selector/1 -> Scope2/1, Heat Trans/2(Surrounding_T)  "<T>"
  Bus Selector/2 -> Heat Trans/3(type)  "<type>"
  Bus Selector1/1 -> Scope3/1, Heat Trans/1(Inner_T)  "<T>"
  Spot T/1 -> Bus Selector1/1
  Surrounding T/1 -> Bus Selector/1

== system model4_2/Thermal point11/Thermal trans3 ==
  Surrounding T : Inport
  Spot T : Inport  Port=2
  Bus Selector : BusSelector  OutputSignals=T,type
  Bus Selector1 : BusSelector  OutputSignals=T
  Heat Trans : MATLAB Function  TreatAsAtomicUnit=on
  Scope : Scope
  Scope2 : Scope
  Scope3 : Scope
  Outer Heat : Outport
  wires:
  Heat Trans/1(Outer_Heat) -> Scope/1, Outer Heat/1
  Bus Selector/1 -> Scope2/1, Heat Trans/2(Surrounding_T)  "<T>"
  Bus Selector/2 -> Heat Trans/3(type)  "<type>"
  Bus Selector1/1 -> Scope3/1, Heat Trans/1(Inner_T)  "<T>"
  Spot T/1 -> Bus Selector1/1
  Surrounding T/1 -> Bus Selector/1

== system model4_2/Thermal point11/Thermal trans4 ==
  Surrounding T : Inport
  Spot T : Inport  Port=2
  Bus Selector : BusSelector  OutputSignals=T,type
  Bus Selector1 : BusSelector  OutputSignals=T
  Heat Trans : MATLAB Function  TreatAsAtomicUnit=on
  Scope : Scope
  Scope2 : Scope
  Scope3 : Scope
  Outer Heat : Outport
  wires:
  Heat Trans/1(Outer_Heat) -> Scope/1, Outer Heat/1
  Bus Selector/1 -> Scope2/1, Heat Trans/2(Surrounding_T)  "<T>"
  Bus Selector/2 -> Heat Trans/3(type)  "<type>"
  Bus Selector1/1 -> Scope3/1, Heat Trans/1(Inner_T)  "<T>"
  Spot T/1 -> Bus Selector1/1
  Surrounding T/1 -> Bus Selector/1

== system model4_2/Thermal point11/Thermal trans7 ==
  Surrounding T : Inport
  Spot T : Inport  Port=2
  Bus Selector : BusSelector  OutputSignals=T,type
  Bus Selector1 : BusSelector  OutputSignals=T
  Heat Trans : MATLAB Function  TreatAsAtomicUnit=on
  Scope : Scope
  Scope2 : Scope
  Scope3 : Scope
  Outer Heat : Outport
  wires:
  Heat Trans/1(Outer_Heat) -> Scope/1, Outer Heat/1
  Bus Selector/1 -> Scope2/1, Heat Trans/2(Surrounding_T)  "<T>"
  Bus Selector1/1 -> Scope3/1, Heat Trans/1(Inner_T)  "<T>"
  Spot T/1 -> Bus Selector1/1
  Surrounding T/1 -> Bus Selector/1
  Bus Selector/2 -> Heat Trans/3(type)  "<type>"

== system model4_2/Thermal point2/Thermal Subsystem ==
  I : Inport
  Outer Heat : Inport  Port=2
  Bus Creator : BusCreator  Inputs=2
  Electrical model : Subsystem
  Heat model : Subsystem
  Parameter : Subsystem
  "T, SOC" : Subsystem
  Unit Delay : UnitDelay  SampleTime=-1  HasFrameUpgradeWarning=on
  cond : Constant  Value=0
  T : Outport
  wires:
  Parameter/2(Non Varing Parameters) -> Electrical model/3(Non Varing Parameters), Heat model/5(Non Varing Parameters)
  "T, SOC"/1(Varing parameters) -> Electrical model/2(Varing parameters), Heat model/4(Varing parameters)
  I/1 -> Heat model/3(I), Electrical model/1(I)
  Electrical model/2(SOC) -> Parameter/2(SOC)
  Electrical model/1(voltage) -> Heat model/2(voltage)
  Parameter/1("T, SOC") -> Heat model/6("T, SOC"), "T, SOC"/1("T, SOC")
  Outer Heat/1 -> Heat model/1(Outer Heat)
  Heat model/1(T) -> Bus Creator/1, Parameter/1(T)
  Bus Creator/1 -> T/1
  cond/1 -> Unit Delay/1  "type"
  Unit Delay/1 -> Bus Creator/2  "type"

== system model4_2/Thermal point2/Thermal trans ==
  Surrounding T : Inport
  Spot T : Inport  Port=2
  Bus Selector : BusSelector  OutputSignals=T,type
  Bus Selector1 : BusSelector  OutputSignals=T
  Heat Trans : MATLAB Function  TreatAsAtomicUnit=on
  Scope : Scope
  Scope2 : Scope
  Scope3 : Scope
  Outer Heat : Outport
  wires:
  Heat Trans/1(Outer_Heat) -> Scope/1, Outer Heat/1
  Bus Selector/1 -> Scope2/1, Heat Trans/2(Surrounding_T)  "<T>"
  Bus Selector/2 -> Heat Trans/3(type)  "<type>"
  Bus Selector1/1 -> Scope3/1, Heat Trans/1(Inner_T)  "<T>"
  Spot T/1 -> Bus Selector1/1
  Surrounding T/1 -> Bus Selector/1

== system model4_2/Thermal point2/Thermal trans1 ==
  Surrounding T : Inport
  Spot T : Inport  Port=2
  Bus Selector : BusSelector  OutputSignals=T,type
  Bus Selector1 : BusSelector  OutputSignals=T
  Heat Trans : MATLAB Function  TreatAsAtomicUnit=on
  Scope : Scope
  Scope2 : Scope
  Scope3 : Scope
  Outer Heat : Outport
  wires:
  Heat Trans/1(Outer_Heat) -> Scope/1, Outer Heat/1
  Bus Selector/1 -> Scope2/1, Heat Trans/2(Surrounding_T)  "<T>"
  Bus Selector/2 -> Heat Trans/3(type)  "<type>"
  Bus Selector1/1 -> Scope3/1, Heat Trans/1(Inner_T)  "<T>"
  Spot T/1 -> Bus Selector1/1
  Surrounding T/1 -> Bus Selector/1

== system model4_2/Thermal point2/Thermal trans2 ==
  Surrounding T : Inport
  Spot T : Inport  Port=2
  Bus Selector : BusSelector  OutputSignals=T,type
  Bus Selector1 : BusSelector  OutputSignals=T
  Heat Trans : MATLAB Function  TreatAsAtomicUnit=on
  Scope : Scope
  Scope2 : Scope
  Scope3 : Scope
  Outer Heat : Outport
  wires:
  Heat Trans/1(Outer_Heat) -> Scope/1, Outer Heat/1
  Bus Selector/1 -> Scope2/1, Heat Trans/2(Surrounding_T)  "<T>"
  Bus Selector/2 -> Heat Trans/3(type)  "<type>"
  Bus Selector1/1 -> Scope3/1, Heat Trans/1(Inner_T)  "<T>"
  Spot T/1 -> Bus Selector1/1
  Surrounding T/1 -> Bus Selector/1

== system model4_2/Thermal point2/Thermal trans3 ==
  Surrounding T : Inport
  Spot T : Inport  Port=2
  Bus Selector : BusSelector  OutputSignals=T,type
  Bus Selector1 : BusSelector  OutputSignals=T
  Heat Trans : MATLAB Function  TreatAsAtomicUnit=on
  Scope : Scope
  Scope2 : Scope
  Scope3 : Scope
  Outer Heat : Outport
  wires:
  Heat Trans/1(Outer_Heat) -> Scope/1, Outer Heat/1
  Bus Selector/1 -> Scope2/1, Heat Trans/2(Surrounding_T)  "<T>"
  Bus Selector/2 -> Heat Trans/3(type)  "<type>"
  Bus Selector1/1 -> Scope3/1, Heat Trans/1(Inner_T)  "<T>"
  Spot T/1 -> Bus Selector1/1
  Surrounding T/1 -> Bus Selector/1

== system model4_2/Thermal point2/Thermal trans4 ==
  Surrounding T : Inport
  Spot T : Inport  Port=2
  Bus Selector : BusSelector  OutputSignals=T,type
  Bus Selector1 : BusSelector  OutputSignals=T
  Heat Trans : MATLAB Function  TreatAsAtomicUnit=on
  Scope : Scope
  Scope2 : Scope
  Scope3 : Scope
  Outer Heat : Outport
  wires:
  Heat Trans/1(Outer_Heat) -> Scope/1, Outer Heat/1
  Bus Selector/1 -> Scope2/1, Heat Trans/2(Surrounding_T)  "<T>"
  Bus Selector/2 -> Heat Trans/3(type)  "<type>"
  Bus Selector1/1 -> Scope3/1, Heat Trans/1(Inner_T)  "<T>"
  Spot T/1 -> Bus Selector1/1
  Surrounding T/1 -> Bus Selector/1

== system model4_2/Thermal point2/Thermal trans7 ==
  Surrounding T : Inport
  Spot T : Inport  Port=2
  Bus Selector : BusSelector  OutputSignals=T,type
  Bus Selector1 : BusSelector  OutputSignals=T
  Heat Trans : MATLAB Function  TreatAsAtomicUnit=on
  Scope : Scope
  Scope2 : Scope
  Scope3 : Scope
  Outer Heat : Outport
  wires:
  Heat Trans/1(Outer_Heat) -> Scope/1, Outer Heat/1
  Bus Selector/1 -> Scope2/1, Heat Trans/2(Surrounding_T)  "<T>"
  Bus Selector1/1 -> Scope3/1, Heat Trans/1(Inner_T)  "<T>"
  Spot T/1 -> Bus Selector1/1
  Surrounding T/1 -> Bus Selector/1
  Bus Selector/2 -> Heat Trans/3(type)  "<type>"

== system model4_2/Thermal point3/Thermal Subsystem ==
  I : Inport
  Outer Heat : Inport  Port=2
  Bus Creator : BusCreator  Inputs=2
  Electrical model : Subsystem
  Heat model : Subsystem
  Parameter : Subsystem
  "T, SOC" : Subsystem
  Unit Delay : UnitDelay  SampleTime=-1  HasFrameUpgradeWarning=on
  cond : Constant  Value=0
  T : Outport
  wires:
  Parameter/2(Non Varing Parameters) -> Electrical model/3(Non Varing Parameters), Heat model/5(Non Varing Parameters)
  "T, SOC"/1(Varing parameters) -> Electrical model/2(Varing parameters), Heat model/4(Varing parameters)
  I/1 -> Heat model/3(I), Electrical model/1(I)
  Electrical model/2(SOC) -> Parameter/2(SOC)
  Electrical model/1(voltage) -> Heat model/2(voltage)
  Parameter/1("T, SOC") -> Heat model/6("T, SOC"), "T, SOC"/1("T, SOC")
  Outer Heat/1 -> Heat model/1(Outer Heat)
  Heat model/1(T) -> Bus Creator/1, Parameter/1(T)
  Bus Creator/1 -> T/1
  cond/1 -> Unit Delay/1  "type"
  Unit Delay/1 -> Bus Creator/2  "type"

== system model4_2/Thermal point3/Thermal trans ==
  Surrounding T : Inport
  Spot T : Inport  Port=2
  Bus Selector : BusSelector  OutputSignals=T,type
  Bus Selector1 : BusSelector  OutputSignals=T
  Heat Trans : MATLAB Function  TreatAsAtomicUnit=on
  Scope : Scope
  Scope2 : Scope
  Scope3 : Scope
  Outer Heat : Outport
  wires:
  Heat Trans/1(Outer_Heat) -> Scope/1, Outer Heat/1
  Bus Selector/1 -> Scope2/1, Heat Trans/2(Surrounding_T)  "<T>"
  Bus Selector/2 -> Heat Trans/3(type)  "<type>"
  Bus Selector1/1 -> Scope3/1, Heat Trans/1(Inner_T)  "<T>"
  Spot T/1 -> Bus Selector1/1
  Surrounding T/1 -> Bus Selector/1

== system model4_2/Thermal point3/Thermal trans1 ==
  Surrounding T : Inport
  Spot T : Inport  Port=2
  Bus Selector : BusSelector  OutputSignals=T,type
  Bus Selector1 : BusSelector  OutputSignals=T
  Heat Trans : MATLAB Function  TreatAsAtomicUnit=on
  Scope : Scope
  Scope2 : Scope
  Scope3 : Scope
  Outer Heat : Outport
  wires:
  Heat Trans/1(Outer_Heat) -> Scope/1, Outer Heat/1
  Bus Selector/1 -> Scope2/1, Heat Trans/2(Surrounding_T)  "<T>"
  Bus Selector/2 -> Heat Trans/3(type)  "<type>"
  Bus Selector1/1 -> Scope3/1, Heat Trans/1(Inner_T)  "<T>"
  Spot T/1 -> Bus Selector1/1
  Surrounding T/1 -> Bus Selector/1

== system model4_2/Thermal point3/Thermal trans2 ==
  Surrounding T : Inport
  Spot T : Inport  Port=2
  Bus Selector : BusSelector  OutputSignals=T,type
  Bus Selector1 : BusSelector  OutputSignals=T
  Heat Trans : MATLAB Function  TreatAsAtomicUnit=on
  Scope : Scope
  Scope2 : Scope
  Scope3 : Scope
  Outer Heat : Outport
  wires:
  Heat Trans/1(Outer_Heat) -> Scope/1, Outer Heat/1
  Bus Selector/1 -> Scope2/1, Heat Trans/2(Surrounding_T)  "<T>"
  Bus Selector/2 -> Heat Trans/3(type)  "<type>"
  Bus Selector1/1 -> Scope3/1, Heat Trans/1(Inner_T)  "<T>"
  Spot T/1 -> Bus Selector1/1
  Surrounding T/1 -> Bus Selector/1

== system model4_2/Thermal point3/Thermal trans3 ==
  Surrounding T : Inport
  Spot T : Inport  Port=2
  Bus Selector : BusSelector  OutputSignals=T,type
  Bus Selector1 : BusSelector  OutputSignals=T
  Heat Trans : MATLAB Function  TreatAsAtomicUnit=on
  Scope : Scope
  Scope2 : Scope
  Scope3 : Scope
  Outer Heat : Outport
  wires:
  Heat Trans/1(Outer_Heat) -> Scope/1, Outer Heat/1
  Bus Selector/1 -> Scope2/1, Heat Trans/2(Surrounding_T)  "<T>"
  Bus Selector/2 -> Heat Trans/3(type)  "<type>"
  Bus Selector1/1 -> Scope3/1, Heat Trans/1(Inner_T)  "<T>"
  Spot T/1 -> Bus Selector1/1
  Surrounding T/1 -> Bus Selector/1

== system model4_2/Thermal point3/Thermal trans4 ==
  Surrounding T : Inport
  Spot T : Inport  Port=2
  Bus Selector : BusSelector  OutputSignals=T,type
  Bus Selector1 : BusSelector  OutputSignals=T
  Heat Trans : MATLAB Function  TreatAsAtomicUnit=on
  Scope : Scope
  Scope2 : Scope
  Scope3 : Scope
  Outer Heat : Outport
  wires:
  Heat Trans/1(Outer_Heat) -> Scope/1, Outer Heat/1
  Bus Selector/1 -> Scope2/1, Heat Trans/2(Surrounding_T)  "<T>"
  Bus Selector/2 -> Heat Trans/3(type)  "<type>"
  Bus Selector1/1 -> Scope3/1, Heat Trans/1(Inner_T)  "<T>"
  Spot T/1 -> Bus Selector1/1
  Surrounding T/1 -> Bus Selector/1

== system model4_2/Thermal point3/Thermal trans7 ==
  Surrounding T : Inport
  Spot T : Inport  Port=2
  Bus Selector : BusSelector  OutputSignals=T,type
  Bus Selector1 : BusSelector  OutputSignals=T
  Heat Trans : MATLAB Function  TreatAsAtomicUnit=on
  Scope : Scope
  Scope2 : Scope
  Scope3 : Scope
  Outer Heat : Outport
  wires:
  Heat Trans/1(Outer_Heat) -> Scope/1, Outer Heat/1
  Bus Selector/1 -> Scope2/1, Heat Trans/2(Surrounding_T)  "<T>"
  Bus Selector1/1 -> Scope3/1, Heat Trans/1(Inner_T)  "<T>"
  Spot T/1 -> Bus Selector1/1
  Surrounding T/1 -> Bus Selector/1
  Bus Selector/2 -> Heat Trans/3(type)  "<type>"

== system model4_2/Thermal point4/Thermal Subsystem ==
  I : Inport
  Outer Heat : Inport  Port=2
  Bus Creator : BusCreator  Inputs=2
  Electrical model : Subsystem
  Heat model : Subsystem
  Parameter : Subsystem
  "T, SOC" : Subsystem
  Unit Delay : UnitDelay  SampleTime=-1  HasFrameUpgradeWarning=on
  cond : Constant  Value=0
  T : Outport
  wires:
  Parameter/2(Non Varing Parameters) -> Electrical model/3(Non Varing Parameters), Heat model/5(Non Varing Parameters)
  "T, SOC"/1(Varing parameters) -> Electrical model/2(Varing parameters), Heat model/4(Varing parameters)
  I/1 -> Heat model/3(I), Electrical model/1(I)
  Electrical model/2(SOC) -> Parameter/2(SOC)
  Electrical model/1(voltage) -> Heat model/2(voltage)
  Parameter/1("T, SOC") -> Heat model/6("T, SOC"), "T, SOC"/1("T, SOC")
  Outer Heat/1 -> Heat model/1(Outer Heat)
  Heat model/1(T) -> Bus Creator/1, Parameter/1(T)
  Bus Creator/1 -> T/1
  cond/1 -> Unit Delay/1  "type"
  Unit Delay/1 -> Bus Creator/2  "type"
